simulink model "sfbuilder_euler2dc"  (Simulink 6.0)
settings: Solver=FixedStepDiscrete  StartTime=0.0  StopTime=10.0  FixedStep=0.020  RelTol=1e-3
libraries: simulink x1
settings Model: Creator=The MathWorks Inc.  LastModifiedBy=batserve  ExtModeAutoUpdateStatusClock=off  ProdHWDeviceType=Specified
settings DataIOCC: SignalLoggingName=sigsOut
settings OptimizationCC: BooleanDataType=off
settings DebuggingCC: CheckExecutionContextPreStartOutputMsg=on  CheckExecutionContextRuntimeOutputMsg=on  SolverPrmCheckMsg=none
settings HardwareCC: ProdHWDeviceType=Specified

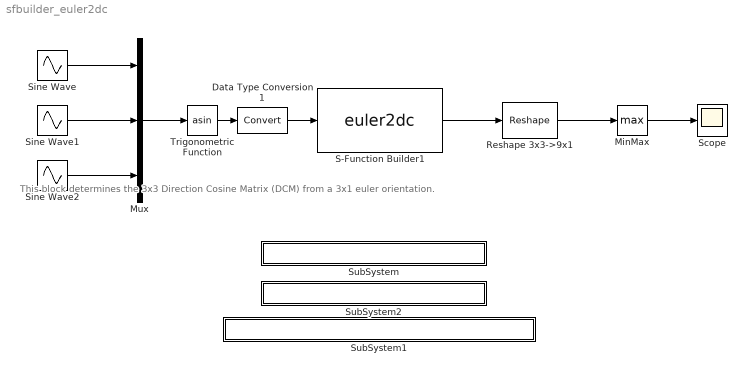
== system sfbuilder_euler2dc ==
  note: This block determines the 3x3 Direction Cosine Matrix (DCM)
      | from a 3x1 euler orientation.
  Data Type Conversion1 : DataTypeConversion  OutDataTypeMode=single  SaturateOnIntegerOverflow=on  RndMeth=Zero
  MinMax : MinMax  Function=max  ZeroCross=off  SaturateOnIntegerOverflow=on  InputSameDT=on
  Mux : Mux  Inputs=3
  Reshape 3x3->9x1 : simulink/Math Operations/Reshape  OutputDimensionality=Column vector  OutputDimensions=[3,3]
  S-Function Builder1 : S-Function  FunctionName=euler2dc  SFunctionModules=euler2dc_wrapper  WizardData=DataTag0  mask(S-Function Builder){}
      mask init:
      | val = [[.9  0.75 0.75 1 1 .9 .9 1]',[1 1 0.75 0.75 .9 .9 1 .9]'];
      | sys = get_param(gcb,'FunctionName');
      settings: CopyFcn=set_param(gcb,'LinkStatus','none')  OpenFcn=sfunctionwizard(gcbh)
      mask Display:
      | plot(val(:,1),val(:,2))
      | disp(sys)
      | port_label('input',1,'worke')
      | port_label('output',1,'dircos')
  Scope : Scope
      settings: TimeRange=10  YMin=0.6  YMax=1
  Sine Wave : Sin  SampleTime=0
  Sine Wave1 : Sin  Phase=1  SampleTime=0
  Sine Wave2 : Sin  Phase=2  SampleTime=0
  SubSystem : Subsystem  PropExecContextAcrossSSBoundary=on
      settings: AttributesFormatString=\n  OpenFcn=edit(fullfile(matlabroot,'simulink','src','euler2dc.c'))
      mask Display: disp('matlabroot\simulink\src\eulerdc.c');
  SubSystem1 : Subsystem  PropExecContextAcrossSSBoundary=on
      settings: AttributesFormatString=\n  OpenFcn=edit(fullfile(matlabroot,'toolbox','simulink','blocks','tlc_c','euler2dc.tlc'))
      mask Display: disp('matlabroot\toolbox\simulink\blocks\tlc_c\euler2dc.tlc');
  SubSystem2 : Subsystem  PropExecContextAcrossSSBoundary=on
      settings: AttributesFormatString=\n\n  OpenFcn=edit(fullfile(matlabroot,'simulink','src','euler2dc_wrapper.c'))
      mask Display: disp('matlabroot\simulink\src\eulerdc_wrapper.c');
  Trigonometric Function : Trigonometry  Operator=asin
  wires:
  Sine Wave/1 -> Mux/1
  Sine Wave1/1 -> Mux/2
  Sine Wave2/1 -> Mux/3
  Mux/1 -> Trigonometric Function/1
  Trigonometric Function/1 -> Data Type Conversion1/1
  S-Function Builder1/1 -> Reshape 3x3->9x1/1
  Reshape 3x3->9x1/1 -> MinMax/1
  Data Type Conversion1/1 -> S-Function Builder1/1
  MinMax/1 -> Scope/1

== system sfbuilder_euler2dc/SubSystem ==

== system sfbuilder_euler2dc/SubSystem1 ==

== system sfbuilder_euler2dc/SubSystem2 ==
